simulink subsystem "ExternalSignalSource"  (R2023b)
settings: Solver=VariableStepAuto  StartTime=0.0  StopTime=10.0  RelTol=1e-3
settings Model: Creator=The MathWorks, Inc.  LastModifiedBy=The MathWorks, Inc.

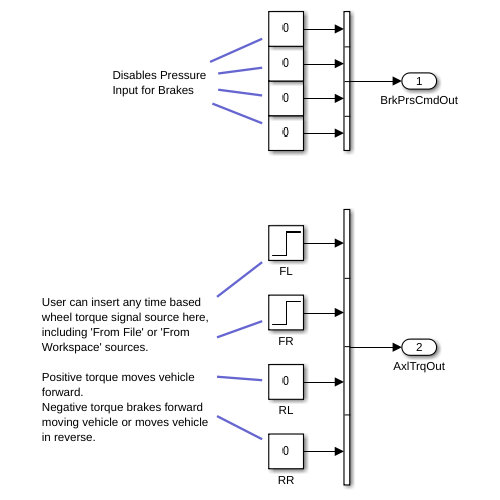
[thumbnail: Simulink's stored preview of the top-level diagram]
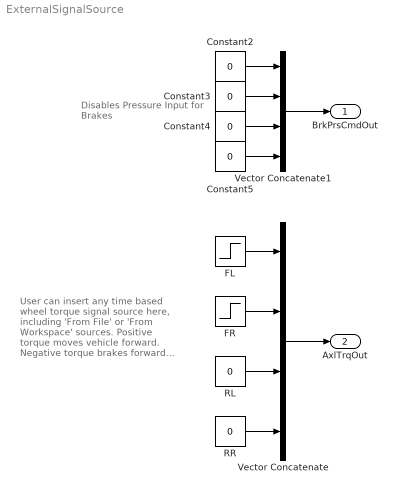
== system ExternalSignalSource ==
  note: Disables Pressure
      | Input for Brakes
  note: User can insert any time based
      | wheel torque signal source here,
      | including 'From File' or 'From
      | Workspace' sources.
      |
      | Positive torque moves vehicle
      | forward.
      | Negative torque brakes forward
      | moving vehicle or moves vehicle
      | in reverse.
  Constant{2..5} (4 alike) : Constant  Value=0  SampleTime=-1
  FL : Step  After=100  SampleTime=0
  FR : Step  After=100  SampleTime=0
  RL : Constant  Value=0  SampleTime=-1
  RR : Constant  Value=0  SampleTime=-1
  Vector Concatenate : Concatenate  NumInputs=4
  Vector Concatenate1 : Concatenate  NumInputs=4
  BrkPrsCmdOut : Outport
  AxlTrqOut : Outport  Port=2
  wires:
  Constant5/1 -> Vector Concatenate1/4
  Vector Concatenate1/1 -> BrkPrsCmdOut/1
  Constant4/1 -> Vector Concatenate1/3
  Constant3/1 -> Vector Concatenate1/2
  Constant2/1 -> Vector Concatenate1/1
  Vector Concatenate/1 -> AxlTrqOut/1
  RR/1 -> Vector Concatenate/4
  RL/1 -> Vector Concatenate/3
  FR/1 -> Vector Concatenate/2
  FL/1 -> Vector Concatenate/1
